simulink model "RiccatiRegler_Anlage"  (R2016b)
settings: Solver=ode1  StartTime=0.0  StopTime=Inf  FixedStep=0.001  RelTol=1e-3
PostLoadFcn:
  | , if any(exist('dsrtsu_mdlpostloadfcn', 'file') == [2, 3, 6]), try dsrtsu_mdlpostloadfcn('Execute', bdroot); catch fprintf('Error in PostLoadFcn (dsrtsu_mdlpostloadfcn) for model "%s":\n %s\n', bdroot, lasterr); end, end,
undefined symbols (not defined in the file): A1k, A2k, Ak, B1, B1k, B2, B2k, Bk, C1k, C2k, Ck, Continuous, K, param, R1k, R2k, Time
libraries: rti1202lib_dac_class1 x3, rti1202lib_adc_class1 x3, simulink_extras x2, ctrlSharedLib x2, rtiemclib x2, simulink x1, rti1202lib_base x1
(part 2 of 2)

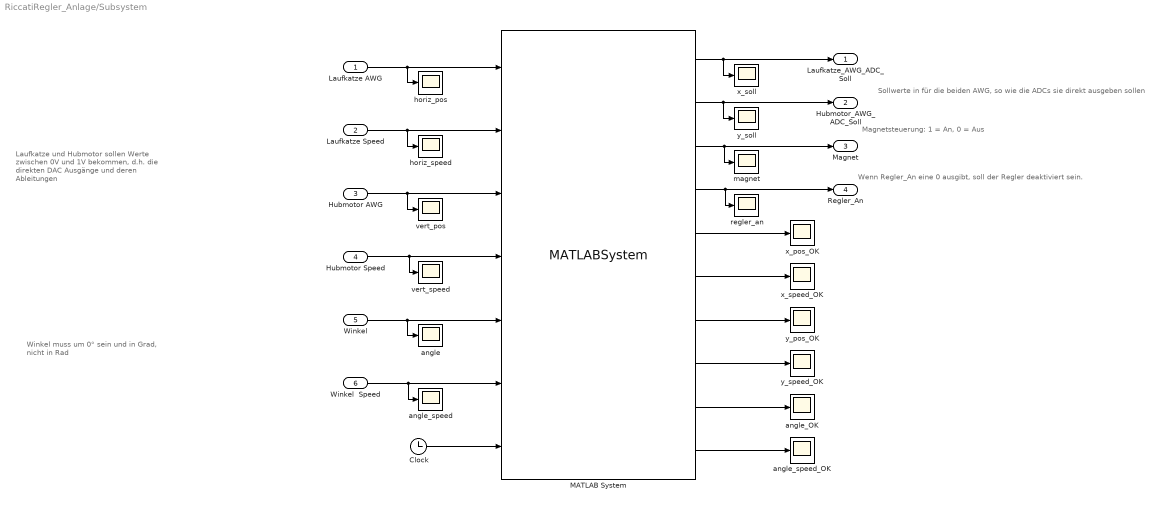
== system RiccatiRegler_Anlage/Subsystem ==
  note: Winkel muss um 0° sein und in Grad,
      | nicht in Rad
  note: Magnetsteuerung: 1 = An, 0 = Aus
  note: Sollwerte in für die beiden AWG, so wie die ADCs sie direkt ausgeben sollen
  note: Wenn Regler_An eine 0 ausgibt, soll der Regler deaktiviert sein.
  note: Laufkatze und Hubmotor sollen
      | Werte zwischen 0V und 1V bekommen,
      | d.h. die direkten DAC Ausgänge und
      | deren Ableitungen
  Laufkatze AWG : Inport  OutMin=0  OutMax=1  OutDataTypeStr=double  PortDimensions=1
  Laufkatze Speed : Inport  Port=2  OutDataTypeStr=double
  Hubmotor AWG : Inport  Port=3  OutMin=0  OutMax=1  OutDataTypeStr=double  PortDimensions=1
  Hubmotor Speed : Inport  Port=4  OutDataTypeStr=double
  Winkel : Inport  Port=5  OutMin=0  OutMax=360  OutDataTypeStr=double  PortDimensions=1
  Winkel  Speed : Inport  Port=6  OutDataTypeStr=double
  Clock : Clock
  MATLAB System : MATLABSystem  System=Steuerung_Automatisierung  start_time=20  add_midpoints=true  midpoint_height=35  param=param  SimulateUsing=Code generation
      mask Type: Steuerung_Automatisierung
      mask Display:
      | disp('Steuerung_Automatisierung');
      | port_label('input',1,'horiz_pos');
      | port_label('input',2,'horiz_speed');
      | port_label('input',3,'vert_pos');
      | port_label('input',4,'vert_speed');
      | port_label('input',5,'angle');
      | port_label('input',6,'angle_speed');
      | port_label('input',7,'Clock');
      | port_label('output',1,'horiz_setpoint');
      | port_label('output',2,'vert_setpoint');
      | port_label('output',3,'magnet_on');
      | port_label('output',4,'control_enable');
      | port_label('output',5,'x_under_thres');
      | port_label('output',6,'x_speed_under_thres');
      | port_label('output',7,'y_under_thres');
      | port_label('output',8,'y_speed_under_thres');
      | port_label('output',9,'angle_under_thres');
      | port_label('output',10,'angle_speed_under_thres');
  angle : Scope
  angle_OK : Scope
  angle_speed : Scope
  angle_speed_OK : Scope
  horiz_pos : Scope
  horiz_speed : Scope
  magnet : Scope
  regler_an : Scope
  vert_pos : Scope
  vert_speed : Scope
  x_pos_OK : Scope
  x_soll : Scope
  x_speed_OK : Scope
  y_pos_OK : Scope
  y_soll : Scope
  y_speed_OK : Scope
  Laufkatze_AWG_ADC_Soll : Outport
  Hubmotor_AWG_ADC_Soll : Outport  Port=2
  Magnet : Outport  Port=3
  Regler_An : Outport  Port=4
  wires:
  Laufkatze AWG/1 -> MATLAB System/1, horiz_pos/1
  Hubmotor AWG/1 -> MATLAB System/3, vert_pos/1
  Winkel/1 -> MATLAB System/5, angle/1
  MATLAB System/4 -> regler_an/1, Regler_An/1
  MATLAB System/1 -> x_soll/1, Laufkatze_AWG_ADC_Soll/1
  MATLAB System/3 -> Magnet/1, magnet/1
  Clock/1 -> MATLAB System/7
  MATLAB System/2 -> y_soll/1, Hubmotor_AWG_ADC_Soll/1
  MATLAB System/5 -> x_pos_OK/1
  MATLAB System/6 -> x_speed_OK/1
  MATLAB System/7 -> y_pos_OK/1
  MATLAB System/8 -> y_speed_OK/1
  MATLAB System/9 -> angle_OK/1
  MATLAB System/10 -> angle_speed_OK/1
  Laufkatze Speed/1 -> MATLAB System/2, horiz_speed/1
  Hubmotor Speed/1 -> MATLAB System/4, vert_speed/1
  Winkel  Speed/1 -> MATLAB System/6, angle_speed/1

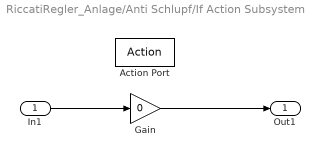
== system RiccatiRegler_Anlage/Anti Schlupf/If Action Subsystem ==
  In1 : Inport
  Action Port : ActionPort  ActionType=then
  Gain : Gain  Gain=0
  Out1 : Outport
  wires:
  In1/1 -> Gain/1
  Gain/1 -> Out1/1

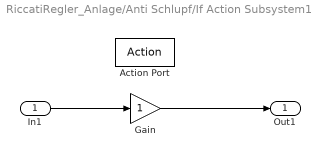
== system RiccatiRegler_Anlage/Anti Schlupf/If Action Subsystem1 ==
  In1 : Inport
  Action Port : ActionPort  ActionType=else
  Gain : Gain
  Out1 : Outport
  wires:
  In1/1 -> Gain/1
  Gain/1 -> Out1/1

== system RiccatiRegler_Anlage/RTI Data/RTI Data Store ==
  RTI Data Store : Subsystem  mask(RTI_DATA_STORE){}
      mask help:
      | RTI Data Store Block. This block is used by RTI to store internal model dependent data. Deleting this block will result in data loss.
      |
      | NEVER DELETE, COPY, OR MODIFY THIS BLOCK!
      mask Help:
      | RTI Data Store Block. This block is used by RTI to store internal model dependent data. Deleting this block will result in data loss.
      | 
      | NEVER DELETE, COPY, OR MODIFY THIS BLOCK!
      mask Display: text(0.5, 0.5, ' ', 'HorizontalAlignment', 'center');

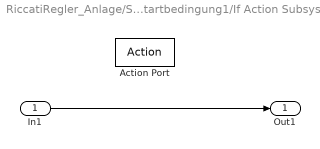
== system RiccatiRegler_Anlage/Startbedingung1/If Action Subsystem ==
  In1 : Inport
  Action Port : ActionPort  InitializeStates=reset  PropagateVarSize=During execution  ActionType=then
  Out1 : Outport
  wires:
  In1/1 -> Out1/1

== system RiccatiRegler_Anlage/Startbedingung2/If Action Subsystem ==
  In1 : Inport
  Action Port : ActionPort  InitializeStates=reset  PropagateVarSize=During execution  ActionType=then
  Out1 : Outport
  wires:
  In1/1 -> Out1/1

== system RiccatiRegler_Anlage/Startbedingung3/If Action Subsystem ==
  In1 : Inport
  Action Port : ActionPort  ActionType=then
  Out1 : Outport
  wires:
  In1/1 -> Out1/1

== system RiccatiRegler_Anlage/Startbedingung4/If Action Subsystem ==
  In1 : Inport
  Action Port : ActionPort  ActionType=then
  Out1 : Outport
  wires:
  In1/1 -> Out1/1

== system RiccatiRegler_Anlage/RTI Data/RTI Data Store/RTI Data Store ==
  RTI Data Store : Subsystem  mask(RTI_DATA_STORE){}
      mask help:
      | RTI Data Store Block. This block is used by RTI to store internal model dependent data. Deleting this block will result in data loss.
      |
      | NEVER DELETE, COPY, OR MODIFY THIS BLOCK!
      mask Help:
      | RTI Data Store Block. This block is used by RTI to store internal model dependent data. Deleting this block will result in data loss.
      | 
      | NEVER DELETE, COPY, OR MODIFY THIS BLOCK!
      mask Display: text(0.5, 0.5, ' ', 'HorizontalAlignment', 'center');

== system RiccatiRegler_Anlage/RTI Data/RTI Data Store/RTI Data Store/RTI Data Store ==
  RTI Data Store : Subsystem  mask(RTI_DATA_STORE){}
      mask help:
      | RTI Data Store Block. This block is used by RTI to store internal model dependent data. Deleting this block will result in data loss.
      |
      | NEVER DELETE, COPY, OR MODIFY THIS BLOCK!
      mask Help:
      | RTI Data Store Block. This block is used by RTI to store internal model dependent data. Deleting this block will result in data loss.
      | 
      | NEVER DELETE, COPY, OR MODIFY THIS BLOCK!
      mask Display: text(0.5, 0.5, ' ', 'HorizontalAlignment', 'center');

== system RiccatiRegler_Anlage/RTI Data/RTI Data Store/RTI Data Store/RTI Data Store/RTI Data Store ==

== matlab function RiccatiRegler_Anlage/Umrechnung Sensor ==
  data: theta_sensor input; theta output
function theta  = sensorWinkel(theta_sensor)
% berechnet aus dem gemessenen Winkel den tatsächlichen Winkel des
% Lasthebers

% l_verb: Länge des Verbindungsstücks
% l_welle: Abstand der beiden Wellen

% Parameter für die Winkelumrechnung
l_verb = 0.109; % m %
l_welle = 0.0575; % m %

theta = asin(sin(theta_sensor) * (l_verb / sqrt(l_welle^2 + l_verb^2 - (2 * l_verb * l_welle * cos(theta_sensor)))));
